simulink library "twiddle_lib"  (Simulink 6.2)
libraries: xbsIndex_r3 x98, coeff_gen_lib x2, twiddle_lib x1
settings Model: LastModifiedBy=aparsons

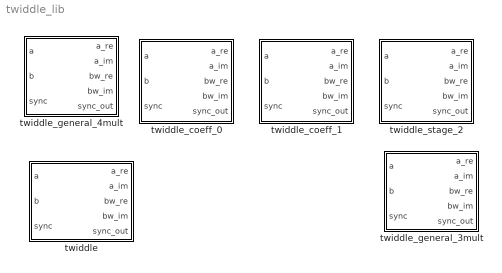
== system twiddle_lib ==
  twiddle : Subsystem  BlockChoice=twiddle_coeff_0
      settings: TemplateBlock=self  MemberBlocks=twiddle_coeff_0,twiddle_coeff_1,twiddle_general_3mult,twiddle_general_4mult,twiddle_stage_2
  twiddle_coeff_0 : Subsystem  mask{BitWidth=18, add_latency=3, mult_latency=4, bram_latency=4}
      mask prompts: BitWidth "Bit Width"; add_latency "Add Latency"; mult_latency "Mult Latency"; bram_latency "BRAM Latency"
      mask init:
      | cursys = gcb;
      | disp(cursys);
  twiddle_coeff_1 : Subsystem  mask{BitWidth=18, add_latency=3, mult_latency=4, bram_latency=4}
      mask prompts: BitWidth "Bit Width"; add_latency "Add Latency"; mult_latency "Mult Latency"; bram_latency "BRAM Latency"
      mask init:
      | cursys = gcb;
      | disp(cursys);
  twiddle_general_3mult : Subsystem  mask{Coeffs=[0], StepPeriod=0, BitWidth=18, add_latency=3, mult_latency=4, bram_latency=4}
      mask prompts: Coeffs "Coefficients:"; StepPeriod "Coefficient Step Period (2^?)"; BitWidth "Bit Width"; add_latency "Add Latency"; mult_latency "Mult Latency"; bram_latency "BRAM Latency"
      mask init:
      | cursys = gcb;
      | disp(cursys);
  twiddle_general_4mult : Subsystem  mask{Coeffs=[0], StepPeriod=0, BitWidth=18, add_latency=3, mult_latency=4, bram_latency=4}
      mask prompts: Coeffs "Coefficients:"; StepPeriod "Coefficient Step Period (2^?)"; BitWidth "Bit Width"; add_latency "Add Latency"; mult_latency "Mult Latency"; bram_latency "BRAM Latency"
      mask init:
      | cursys = gcb;
      | disp(cursys);
  twiddle_stage_2 : Subsystem  mask{FFTSize=5, BitWidth=18, add_latency=3, mult_latency=4, bram_latency=4}
      mask prompts: FFTSize "Size of FFT: (2^?)"; BitWidth "Bit Width"; add_latency "Add Latency"; mult_latency "Mult Latency"; bram_latency "BRAM Latency"
      mask init:
      | cursys = gcb;
      | disp(cursys);

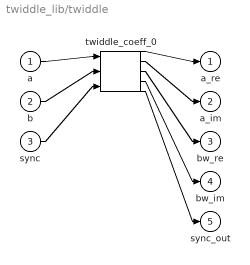
== system twiddle_lib/twiddle ==
  a : Inport  Port=1  LatchInput=off
  b : Inport  Port=2  LatchInput=off
  sync : Inport  Port=3  LatchInput=off
  twiddle_coeff_0 : twiddle_lib/twiddle_coeff_0  BitWidth=18  add_latency=3  mult_latency=4  bram_latency=4
  a_re : Outport
  a_im : Outport  Port=2
  bw_re : Outport  Port=3
  bw_im : Outport  Port=4
  sync_out : Outport  Port=5
  wires:
  a/1 -> twiddle_coeff_0/1
  b/1 -> twiddle_coeff_0/2
  sync/1 -> twiddle_coeff_0/3
  twiddle_coeff_0/1 -> a_re/1
  twiddle_coeff_0/2 -> a_im/1
  twiddle_coeff_0/3 -> bw_re/1
  twiddle_coeff_0/4 -> bw_im/1
  twiddle_coeff_0/5 -> sync_out/1

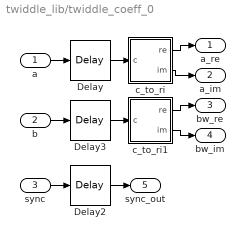
== system twiddle_lib/twiddle_coeff_0 ==
  a : Inport  Port=1  LatchInput=off
  b : Inport  Port=2  LatchInput=off
  sync : Inport  Port=3  LatchInput=off
  Delay : xbsIndex_r3/Delay  latency=mult_latency + add_latency + bram_latency  reg_retiming=off  explicit_period=off  period=1  en=off  accept_only_valid=off  init_zero=on  dbl_ovrd=off  show_param=off
      settings: xl_area=[0, 0, 0, 0, 0, 0, 0]
  Delay2 : xbsIndex_r3/Delay  latency=mult_latency + add_latency + bram_latency  reg_retiming=off  explicit_period=off  period=1  en=off  accept_only_valid=off  init_zero=on  dbl_ovrd=off  show_param=off
      settings: xl_area=[0, 0, 0, 0, 0, 0, 0]
  Delay3 : xbsIndex_r3/Delay  latency=mult_latency + add_latency + bram_latency  reg_retiming=off  explicit_period=off  period=1  en=off  accept_only_valid=off  init_zero=on  dbl_ovrd=off  show_param=off
      settings: xl_area=[0, 0, 0, 0, 0, 0, 0]
  c_to_ri : Subsystem
  c_to_ri1 : Subsystem
  a_re : Outport
  a_im : Outport  Port=2
  bw_re : Outport  Port=3
  bw_im : Outport  Port=4
  sync_out : Outport  Port=5
  wires:
  Delay3/1 -> c_to_ri1/1(c)
  c_to_ri1/2(im) -> bw_im/1
  c_to_ri1/1(re) -> bw_re/1
  c_to_ri/2(im) -> a_im/1
  c_to_ri/1(re) -> a_re/1
  Delay/1 -> c_to_ri/1(c)
  b/1 -> Delay3/1
  Delay2/1 -> sync_out/1
  sync/1 -> Delay2/1
  a/1 -> Delay/1

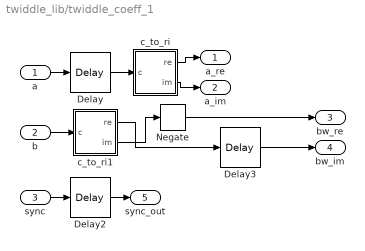
== system twiddle_lib/twiddle_coeff_1 ==
  a : Inport  Port=1  LatchInput=off
  b : Inport  Port=2  LatchInput=off
  sync : Inport  Port=3  LatchInput=off
  Delay : xbsIndex_r3/Delay  latency=mult_latency + add_latency + bram_latency  reg_retiming=off  explicit_period=off  period=1  en=off  accept_only_valid=off  init_zero=on  dbl_ovrd=off  show_param=off
      settings: xl_area=[0, 0, 0, 0, 0, 0, 0]
  Delay2 : xbsIndex_r3/Delay  latency=mult_latency + add_latency + bram_latency  reg_retiming=off  explicit_period=off  period=1  en=off  accept_only_valid=off  init_zero=on  dbl_ovrd=off  show_param=off
      settings: xl_area=[0, 0, 0, 0, 0, 0, 0]
  Delay3 : xbsIndex_r3/Delay  latency=mult_latency + add_latency + bram_latency  reg_retiming=off  explicit_period=off  period=1  en=off  accept_only_valid=off  init_zero=on  dbl_ovrd=off  show_param=off
      settings: xl_area=[0, 0, 0, 0, 0, 0, 0]
  Negate : xbsIndex_r3/Negate  precision=User Defined  arith_type="Signed  (2's comp)"  n_bits=BitWidth  bin_pt=BitWidth-1  quantization=Truncate  overflow=Wrap  latency=mult_latency + add_latency + bram_latency  explicit_period=off  period=1  en=off  dbl_ovrd=off  use_core=on  show_param=off  use_rpm=on  gen_core=off
      settings: xl_area=[0, 0, 0, 0, 0, 0, 0]
  c_to_ri : Subsystem
  c_to_ri1 : Subsystem
  a_re : Outport
  a_im : Outport  Port=2
  bw_re : Outport  Port=3
  bw_im : Outport  Port=4
  sync_out : Outport  Port=5
  wires:
  Delay3/1 -> bw_im/1
  c_to_ri1/2(im) -> Negate/1
  Negate/1 -> bw_re/1
  c_to_ri1/1(re) -> Delay3/1
  a/1 -> Delay/1
  sync/1 -> Delay2/1
  Delay2/1 -> sync_out/1
  b/1 -> c_to_ri1/1(c)
  Delay/1 -> c_to_ri/1(c)
  c_to_ri/1(re) -> a_re/1
  c_to_ri/2(im) -> a_im/1

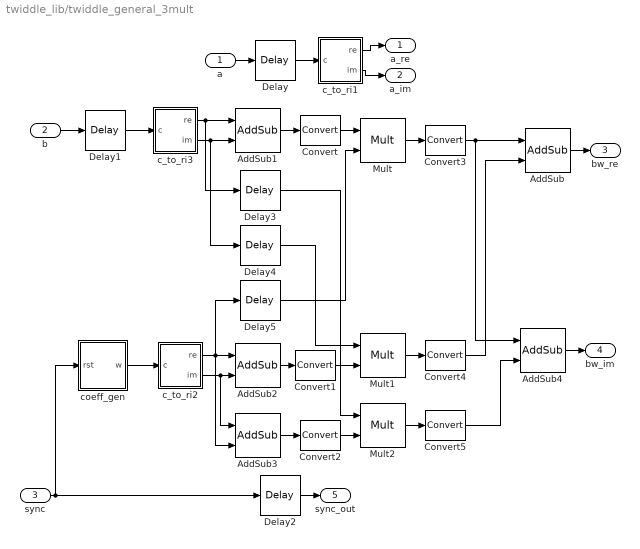
== system twiddle_lib/twiddle_general_3mult ==
  a : Inport  Port=1  LatchInput=off
  b : Inport  Port=2  LatchInput=off
  sync : Inport  Port=3  LatchInput=off
  AddSub : xbsIndex_r3/AddSub  mode=Subtraction  precision=Full  arith_type="Signed  (2's comp)"  n_bits=BitWidth  bin_pt=BitWidth - 1  quantization="Round  (unbiased: +/- Inf)"  overflow=Wrap  latency=add_latency  explicit_period=off  period=1  use_carryin=off  use_carryout=off  en=off  dbl_ovrd=off  show_param=on  use_core=on  pipeline=on  use_rpm=on  gen_core=on
      settings: xl_area=[0, 0, 0, 0, 0, 0, 0]
  AddSub1 : xbsIndex_r3/AddSub  mode=Addition  precision=Full  arith_type="Signed  (2's comp)"  n_bits=BitWidth  bin_pt=BitWidth - 1  quantization="Round  (unbiased: +/- Inf)"  overflow=Wrap  latency=add_latency  explicit_period=off  period=1  use_carryin=off  use_carryout=off  en=off  dbl_ovrd=off  show_param=on  use_core=on  pipeline=on  use_rpm=on  gen_core=on
      settings: xl_area=[0, 0, 0, 0, 0, 0, 0]
  AddSub2 : xbsIndex_r3/AddSub  mode=Addition  precision=Full  arith_type="Signed  (2's comp)"  n_bits=BitWidth  bin_pt=BitWidth - 1  quantization="Round  (unbiased: +/- Inf)"  overflow=Wrap  latency=add_latency  explicit_period=off  period=1  use_carryin=off  use_carryout=off  en=off  dbl_ovrd=off  show_param=on  use_core=on  pipeline=on  use_rpm=on  gen_core=on
      settings: xl_area=[0, 0, 0, 0, 0, 0, 0]
  AddSub3 : xbsIndex_r3/AddSub  mode=Subtraction  precision=Full  arith_type="Signed  (2's comp)"  n_bits=BitWidth  bin_pt=BitWidth - 1  quantization="Round  (unbiased: +/- Inf)"  overflow=Wrap  latency=add_latency  explicit_period=off  period=1  use_carryin=off  use_carryout=off  en=off  dbl_ovrd=off  show_param=on  use_core=on  pipeline=on  use_rpm=on  gen_core=on
      settings: xl_area=[0, 0, 0, 0, 0, 0, 0]
  AddSub4 : xbsIndex_r3/AddSub  mode=Addition  precision=Full  arith_type="Signed  (2's comp)"  n_bits=BitWidth  bin_pt=BitWidth - 1  quantization="Round  (unbiased: +/- Inf)"  overflow=Wrap  latency=add_latency  explicit_period=off  period=1  use_carryin=off  use_carryout=off  en=off  dbl_ovrd=off  show_param=on  use_core=on  pipeline=on  use_rpm=on  gen_core=on
      settings: xl_area=[0, 0, 0, 0, 0, 0, 0]
  Convert : xbsIndex_r3/Convert  arith_type="Signed  (2's comp)"  n_bits=BitWidth  bin_pt=BitWidth-2  quantization=Truncate  overflow=Wrap  latency=0  explicit_period=off  period=1  dbl_ovrd=off  show_param=off  inserted_by_tool=off  pipeline=off
      settings: xl_area=[0, 0, 0, 0, 0, 0, 0]
  Convert1 : xbsIndex_r3/Convert  arith_type="Signed  (2's comp)"  n_bits=BitWidth  bin_pt=BitWidth-2  quantization=Truncate  overflow=Wrap  latency=0  explicit_period=off  period=1  dbl_ovrd=off  show_param=off  inserted_by_tool=off  pipeline=off
      settings: xl_area=[0, 0, 0, 0, 0, 0, 0]
  Convert2 : xbsIndex_r3/Convert  arith_type="Signed  (2's comp)"  n_bits=BitWidth  bin_pt=BitWidth-2  quantization=Truncate  overflow=Wrap  latency=0  explicit_period=off  period=1  dbl_ovrd=off  show_param=off  inserted_by_tool=off  pipeline=off
      settings: xl_area=[0, 0, 0, 0, 0, 0, 0]
  Convert3 : xbsIndex_r3/Convert  arith_type="Signed  (2's comp)"  n_bits=BitWidth + 3  bin_pt=BitWidth  quantization=Truncate  overflow=Wrap  latency=0  explicit_period=off  period=1  dbl_ovrd=off  show_param=off  inserted_by_tool=off  pipeline=off
      settings: xl_area=[0, 0, 0, 0, 0, 0, 0]
  Convert4 : xbsIndex_r3/Convert  arith_type="Signed  (2's comp)"  n_bits=BitWidth + 3  bin_pt=BitWidth  quantization=Truncate  overflow=Wrap  latency=0  explicit_period=off  period=1  dbl_ovrd=off  show_param=off  inserted_by_tool=off  pipeline=off
      settings: xl_area=[0, 0, 0, 0, 0, 0, 0]
  Convert5 : xbsIndex_r3/Convert  arith_type="Signed  (2's comp)"  n_bits=BitWidth + 3  bin_pt=BitWidth  quantization=Truncate  overflow=Wrap  latency=0  explicit_period=off  period=1  dbl_ovrd=off  show_param=off  inserted_by_tool=off  pipeline=off
      settings: xl_area=[0, 0, 0, 0, 0, 0, 0]
  Delay : xbsIndex_r3/Delay  latency=mult_latency + 2*add_latency + bram_latency  reg_retiming=off  explicit_period=off  period=1  en=off  accept_only_valid=off  init_zero=on  dbl_ovrd=off  show_param=off
      settings: xl_area=[0, 0, 0, 0, 0, 0, 0]
  Delay1 : xbsIndex_r3/Delay  latency=bram_latency  reg_retiming=off  explicit_period=off  period=1  en=off  accept_only_valid=off  init_zero=on  dbl_ovrd=off  show_param=off
      settings: xl_area=[0, 0, 0, 0, 0, 0, 0]
  Delay2 : xbsIndex_r3/Delay  latency=mult_latency + 2*add_latency + bram_latency  reg_retiming=off  explicit_period=off  period=1  en=off  accept_only_valid=off  init_zero=on  dbl_ovrd=off  show_param=off
      settings: xl_area=[0, 0, 0, 0, 0, 0, 0]
  Delay3 : xbsIndex_r3/Delay  latency=add_latency  reg_retiming=off  explicit_period=off  period=1  en=off  accept_only_valid=off  init_zero=on  dbl_ovrd=off  show_param=off
      settings: xl_area=[0, 0, 0, 0, 0, 0, 0]
  Delay4 : xbsIndex_r3/Delay  latency=add_latency  reg_retiming=off  explicit_period=off  period=1  en=off  accept_only_valid=off  init_zero=on  dbl_ovrd=off  show_param=off
      settings: xl_area=[0, 0, 0, 0, 0, 0, 0]
  Delay5 : xbsIndex_r3/Delay  latency=add_latency  reg_retiming=off  explicit_period=off  period=1  en=off  accept_only_valid=off  init_zero=on  dbl_ovrd=off  show_param=off
      settings: xl_area=[0, 0, 0, 0, 0, 0, 0]
  Mult : xbsIndex_r3/Mult  precision=Full  arith_type="Signed  (2's comp)"  n_bits=BitWidth  bin_pt=BitWidth-1  quantization="Round  (unbiased: +/- Inf)"  overflow=Wrap  latency=mult_latency  explicit_period=off  period=1  en=off  dbl_ovrd=off  show_param=on  mult_type=Parallel  oversample=2  use_embedded=on  pipeline=on  use_rpm=on  placement_style=Rectangular Shape  gen_core=on
      settings: xl_area=[0, 0, 0, 0, 0, 0, 0]
  Mult1 : xbsIndex_r3/Mult  precision=Full  arith_type="Signed  (2's comp)"  n_bits=BitWidth  bin_pt=BitWidth-1  quantization="Round  (unbiased: +/- Inf)"  overflow=Wrap  latency=mult_latency  explicit_period=off  period=1  en=off  dbl_ovrd=off  show_param=on  mult_type=Parallel  oversample=2  use_embedded=on  pipeline=on  use_rpm=on  placement_style=Rectangular Shape  gen_core=on
      settings: xl_area=[0, 0, 0, 0, 0, 0, 0]
  Mult2 : xbsIndex_r3/Mult  precision=Full  arith_type="Signed  (2's comp)"  n_bits=BitWidth  bin_pt=BitWidth-1  quantization="Round  (unbiased: +/- Inf)"  overflow=Wrap  latency=mult_latency  explicit_period=off  period=1  en=off  dbl_ovrd=off  show_param=on  mult_type=Parallel  oversample=2  use_embedded=on  pipeline=on  use_rpm=on  placement_style=Rectangular Shape  gen_core=on
      settings: xl_area=[0, 0, 0, 0, 0, 0, 0]
  c_to_ri1 : Subsystem
  c_to_ri2 : Subsystem
  c_to_ri3 : Subsystem
  coeff_gen : Subsystem  BlockChoice=static_coeff_gen
      link override br_coeff_gen: Coeffs=Coeffs  StepPeriod=StepPeriod  n_bits=BitWidth  latency=bram_latency
      link override static_coeff_gen: Coeffs=Coeffs  n_bits=BitWidth  latency=bram_latency
      settings: AttributesFormatString=%<BlockChoice>  TemplateBlock=coeff_gen_lib/coeff_gen  MemberBlocks=br_coeff_gen,static_coeff_gen
  a_re : Outport
  a_im : Outport  Port=2
  bw_re : Outport  Port=3
  bw_im : Outport  Port=4
  sync_out : Outport  Port=5
  wires:
  Delay2/1 -> sync_out/1
  sync/1 -> coeff_gen/1(rst), Delay2/1
  a/1 -> Delay/1
  Delay/1 -> c_to_ri1/1(c)
  c_to_ri1/1(re) -> a_re/1
  c_to_ri1/2(im) -> a_im/1
  b/1 -> Delay1/1
  Delay1/1 -> c_to_ri3/1(c)
  coeff_gen/1(w) -> c_to_ri2/1(c)
  c_to_ri3/1(re) -> AddSub1/1, Delay3/1
  c_to_ri3/2(im) -> AddSub1/2, Delay4/1
  c_to_ri2/1(re) -> AddSub2/1, AddSub3/2, Delay5/1
  c_to_ri2/2(im) -> AddSub2/2, AddSub3/1
  AddSub3/1 -> Convert2/1
  AddSub2/1 -> Convert1/1
  AddSub1/1 -> Convert/1
  Convert/1 -> Mult/1
  Convert1/1 -> Mult1/2
  Convert2/1 -> Mult2/2
  Delay4/1 -> Mult1/1
  Delay5/1 -> Mult/2
  Delay3/1 -> Mult2/1
  Mult/1 -> Convert3/1
  Mult1/1 -> Convert4/1
  Mult2/1 -> Convert5/1
  AddSub/1 -> bw_re/1
  AddSub4/1 -> bw_im/1
  Convert3/1 -> AddSub/1, AddSub4/1
  Convert4/1 -> AddSub/2
  Convert5/1 -> AddSub4/2

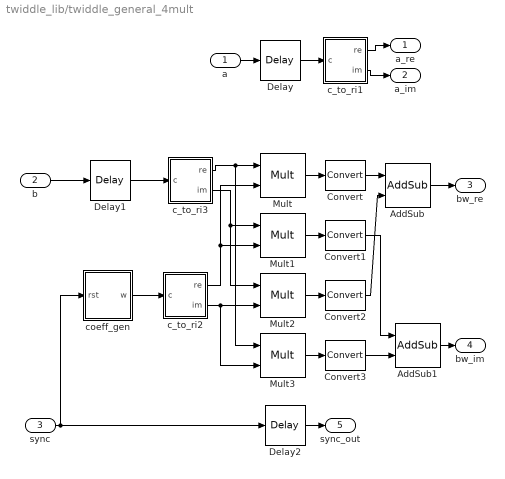
== system twiddle_lib/twiddle_general_4mult ==
  a : Inport  Port=1  LatchInput=off
  b : Inport  Port=2  LatchInput=off
  sync : Inport  Port=3  LatchInput=off
  AddSub : xbsIndex_r3/AddSub  mode=Subtraction  precision=Full  arith_type="Signed  (2's comp)"  n_bits=BitWidth  bin_pt=BitWidth - 1  quantization="Round  (unbiased: +/- Inf)"  overflow=Wrap  latency=add_latency  explicit_period=off  period=1  use_carryin=off  use_carryout=off  en=off  dbl_ovrd=off  show_param=on  use_core=on  pipeline=on  use_rpm=on  gen_core=on
      settings: xl_area=[0, 0, 0, 0, 0, 0, 0]
  AddSub1 : xbsIndex_r3/AddSub  mode=Addition  precision=Full  arith_type="Signed  (2's comp)"  n_bits=BitWidth  bin_pt=BitWidth-1  quantization="Round  (unbiased: +/- Inf)"  overflow=Wrap  latency=add_latency  explicit_period=off  period=1  use_carryin=off  use_carryout=off  en=off  dbl_ovrd=off  show_param=on  use_core=on  pipeline=on  use_rpm=on  gen_core=on
      settings: xl_area=[0, 0, 0, 0, 0, 0, 0]
  Convert{,1..3} (4 alike) : xbsIndex_r3/Convert  arith_type="Signed  (2's comp)"  n_bits=BitWidth + 2  bin_pt=BitWidth  quantization="Round  (unbiased: Even Values)"  overflow=Wrap  latency=0  explicit_period=off  period=1  dbl_ovrd=off  show_param=off  inserted_by_tool=off  pipeline=off
      settings: xl_area=[0, 0, 0, 0, 0, 0, 0]
  Delay : xbsIndex_r3/Delay  latency=mult_latency + add_latency + bram_latency  reg_retiming=off  explicit_period=off  period=1  en=off  accept_only_valid=off  init_zero=on  dbl_ovrd=off  show_param=off
      settings: xl_area=[0, 0, 0, 0, 0, 0, 0]
  Delay1 : xbsIndex_r3/Delay  latency=bram_latency  reg_retiming=off  explicit_period=off  period=1  en=off  accept_only_valid=off  init_zero=on  dbl_ovrd=off  show_param=off
      settings: xl_area=[0, 0, 0, 0, 0, 0, 0]
  Delay2 : xbsIndex_r3/Delay  latency=mult_latency + add_latency + bram_latency  reg_retiming=off  explicit_period=off  period=1  en=off  accept_only_valid=off  init_zero=on  dbl_ovrd=off  show_param=off
      settings: xl_area=[0, 0, 0, 0, 0, 0, 0]
  Mult{,1..3} (4 alike) : xbsIndex_r3/Mult  precision=Full  arith_type="Signed  (2's comp)"  n_bits=BitWidth  bin_pt=BitWidth-1  quantization="Round  (unbiased: +/- Inf)"  overflow=Wrap  latency=mult_latency  explicit_period=off  period=1  en=off  dbl_ovrd=off  show_param=on  mult_type=Parallel  oversample=2  use_embedded=on  pipeline=on  use_rpm=on  placement_style=Rectangular Shape  gen_core=on
      settings: xl_area=[0, 0, 0, 0, 0, 0, 0]
  c_to_ri1 : Subsystem
  c_to_ri2 : Subsystem
  c_to_ri3 : Subsystem
  coeff_gen : Subsystem  BlockChoice=static_coeff_gen
      link override br_coeff_gen: Coeffs=Coeffs  StepPeriod=StepPeriod  n_bits=BitWidth  latency=bram_latency
      link override static_coeff_gen: Coeffs=Coeffs  n_bits=BitWidth  latency=bram_latency
      settings: AttributesFormatString=%<BlockChoice>  TemplateBlock=coeff_gen_lib/coeff_gen  MemberBlocks=br_coeff_gen,static_coeff_gen
  a_re : Outport
  a_im : Outport  Port=2
  bw_re : Outport  Port=3
  bw_im : Outport  Port=4
  sync_out : Outport  Port=5
  wires:
  coeff_gen/1(w) -> c_to_ri2/1(c)
  Delay1/1 -> c_to_ri3/1(c)
  c_to_ri2/2(im) -> Mult3/2, Mult2/2
  c_to_ri3/2(im) -> Mult1/1, Mult2/1
  c_to_ri3/1(re) -> Mult3/1, Mult/1
  b/1 -> Delay1/1
  c_to_ri1/2(im) -> a_im/1
  c_to_ri1/1(re) -> a_re/1
  Delay/1 -> c_to_ri1/1(c)
  AddSub/1 -> bw_re/1
  AddSub1/1 -> bw_im/1
  c_to_ri2/1(re) -> Mult/2, Mult1/2
  Mult/1 -> Convert/1
  Mult2/1 -> Convert2/1
  Mult1/1 -> Convert1/1
  Mult3/1 -> Convert3/1
  a/1 -> Delay/1
  sync/1 -> Delay2/1, coeff_gen/1(rst)
  Delay2/1 -> sync_out/1
  Convert/1 -> AddSub/1
  Convert1/1 -> AddSub1/1
  Convert2/1 -> AddSub/2
  Convert3/1 -> AddSub1/2

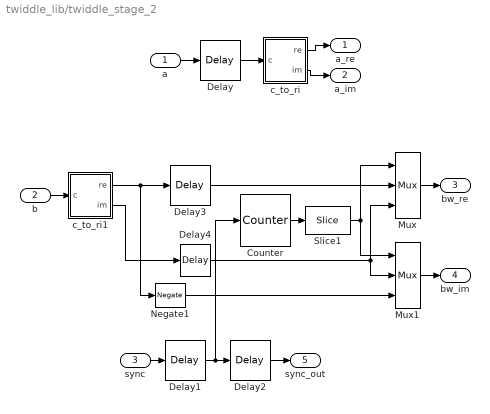
== system twiddle_lib/twiddle_stage_2 ==
  a : Inport  Port=1  LatchInput=off
  b : Inport  Port=2  LatchInput=off
  sync : Inport  Port=3  LatchInput=off
  Counter : xbsIndex_r3/Counter  cnt_type=Free Running  n_bits=FFTSize - 1  bin_pt=0  arith_type=Unsigned  start_count=0  cnt_to=Inf  cnt_by_val=1  operation=Up  explicit_period=off  period=1  load_pin=off  rst=on  en=off  dbl_ovrd=off  show_param=off  use_rpm=on  gen_core=off
      settings: xl_area=[0, 0, 0, 0, 0, 0, 0]
  Delay : xbsIndex_r3/Delay  latency=mult_latency + add_latency + bram_latency  reg_retiming=off  explicit_period=off  period=1  en=off  accept_only_valid=off  init_zero=on  dbl_ovrd=off  show_param=off
      settings: xl_area=[0, 0, 0, 0, 0, 0, 0]
  Delay1 : xbsIndex_r3/Delay  latency=bram_latency  reg_retiming=off  explicit_period=off  period=1  en=off  accept_only_valid=off  init_zero=on  dbl_ovrd=off  show_param=off
      settings: xl_area=[0, 0, 0, 0, 0, 0, 0]
  Delay2 : xbsIndex_r3/Delay  latency=mult_latency + add_latency  reg_retiming=off  explicit_period=off  period=1  en=off  accept_only_valid=off  init_zero=on  dbl_ovrd=off  show_param=off
      settings: xl_area=[0, 0, 0, 0, 0, 0, 0]
  Delay3 : xbsIndex_r3/Delay  latency=bram_latency  reg_retiming=off  explicit_period=off  period=1  en=off  accept_only_valid=off  init_zero=on  dbl_ovrd=off  show_param=off
      settings: xl_area=[0, 0, 0, 0, 0, 0, 0]
  Delay4 : xbsIndex_r3/Delay  latency=bram_latency  reg_retiming=off  explicit_period=off  period=1  en=off  accept_only_valid=off  init_zero=on  dbl_ovrd=off  show_param=off
      settings: xl_area=[0, 0, 0, 0, 0, 0, 0]
  Mux : xbsIndex_r3/Mux  inputs=2  precision=Full  arith_type="Signed  (2's comp)"  n_bits=8  bin_pt=2  quantization=Truncate  overflow=Wrap  latency=mult_latency + add_latency  explicit_period=off  period=1  en=off  dbl_ovrd=off  show_param=off  mux_type=off  use_rpm=off  gen_core=off
      settings: xl_area=[0, 0, 0, 0, 0, 0, 0]
  Mux1 : xbsIndex_r3/Mux  inputs=2  precision=Full  arith_type="Signed  (2's comp)"  n_bits=8  bin_pt=2  quantization=Truncate  overflow=Wrap  latency=mult_latency + add_latency  explicit_period=off  period=1  en=off  dbl_ovrd=off  show_param=off  mux_type=off  use_rpm=off  gen_core=off
      settings: xl_area=[0, 0, 0, 0, 0, 0, 0]
  Negate1 : xbsIndex_r3/Negate  precision=User Defined  arith_type="Signed  (2's comp)"  n_bits=BitWidth  bin_pt=BitWidth-1  quantization=Truncate  overflow=Wrap  latency=bram_latency  explicit_period=off  period=1  en=off  dbl_ovrd=off  use_core=on  show_param=off  use_rpm=on  gen_core=off
      settings: xl_area=[0, 0, 0, 0, 0, 0, 0]
  Slice1 : xbsIndex_r3/Slice  mode=Upper Bit Location + Width  nbits=1  bit1=0  base1=MSB of Input  bit0=0  base0=LSB of Input  boolean_output=off  explicit_period=off  period=1  dbl_ovrd=off
  c_to_ri : Subsystem
  c_to_ri1 : Subsystem
  a_re : Outport
  a_im : Outport  Port=2
  bw_re : Outport  Port=3
  bw_im : Outport  Port=4
  sync_out : Outport  Port=5
  wires:
  Delay4/1 -> Mux/3, Mux1/2
  Delay3/1 -> Mux/2
  Delay1/1 -> Counter/1, Delay2/1
  Mux1/1 -> bw_im/1
  Mux/1 -> bw_re/1
  c_to_ri1/1(re) -> Delay3/1, Negate1/1
  Slice1/1 -> Mux1/1, Mux/1
  Counter/1 -> Slice1/1
  Negate1/1 -> Mux1/3
  c_to_ri1/2(im) -> Delay4/1
  c_to_ri/2(im) -> a_im/1
  c_to_ri/1(re) -> a_re/1
  Delay/1 -> c_to_ri/1(c)
  b/1 -> c_to_ri1/1(c)
  Delay2/1 -> sync_out/1
  sync/1 -> Delay1/1
  a/1 -> Delay/1

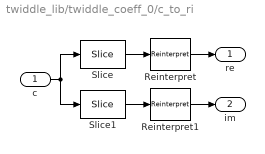
== system twiddle_lib/twiddle_coeff_0/c_to_ri ==
  c : Inport  Port=1  LatchInput=off
  Reinterpret : xbsIndex_r3/Reinterpret  force_arith_type=on  arith_type="Signed  (2's comp)"  force_bin_pt=on  bin_pt=BitWidth - 1  force_valid=on
  Reinterpret1 : xbsIndex_r3/Reinterpret  force_arith_type=on  arith_type="Signed  (2's comp)"  force_bin_pt=on  bin_pt=BitWidth - 1  force_valid=on
  Slice : xbsIndex_r3/Slice  mode=Upper Bit Location + Width  nbits=BitWidth  bit1=0  base1=MSB of Input  bit0=0  base0=LSB of Input  boolean_output=off  explicit_period=off  period=1  dbl_ovrd=off
  Slice1 : xbsIndex_r3/Slice  mode=Lower Bit Location + Width  nbits=BitWidth  bit1=0  base1=MSB of Input  bit0=0  base0=LSB of Input  boolean_output=off  explicit_period=off  period=1  dbl_ovrd=off
  re : Outport
  im : Outport  Port=2
  wires:
  c/1 -> Slice1/1, Slice/1
  Reinterpret1/1 -> im/1
  Reinterpret/1 -> re/1
  Slice1/1 -> Reinterpret1/1
  Slice/1 -> Reinterpret/1

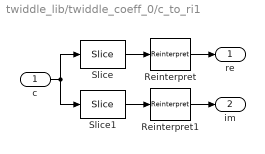
== system twiddle_lib/twiddle_coeff_0/c_to_ri1 ==
  c : Inport  Port=1  LatchInput=off
  Reinterpret : xbsIndex_r3/Reinterpret  force_arith_type=on  arith_type="Signed  (2's comp)"  force_bin_pt=on  bin_pt=BitWidth - 1  force_valid=on
  Reinterpret1 : xbsIndex_r3/Reinterpret  force_arith_type=on  arith_type="Signed  (2's comp)"  force_bin_pt=on  bin_pt=BitWidth - 1  force_valid=on
  Slice : xbsIndex_r3/Slice  mode=Upper Bit Location + Width  nbits=BitWidth  bit1=0  base1=MSB of Input  bit0=0  base0=LSB of Input  boolean_output=off  explicit_period=off  period=1  dbl_ovrd=off
  Slice1 : xbsIndex_r3/Slice  mode=Lower Bit Location + Width  nbits=BitWidth  bit1=0  base1=MSB of Input  bit0=0  base0=LSB of Input  boolean_output=off  explicit_period=off  period=1  dbl_ovrd=off
  re : Outport
  im : Outport  Port=2
  wires:
  c/1 -> Slice1/1, Slice/1
  Reinterpret1/1 -> im/1
  Reinterpret/1 -> re/1
  Slice1/1 -> Reinterpret1/1
  Slice/1 -> Reinterpret/1

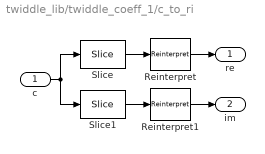
== system twiddle_lib/twiddle_coeff_1/c_to_ri ==
  c : Inport  Port=1  LatchInput=off
  Reinterpret : xbsIndex_r3/Reinterpret  force_arith_type=on  arith_type="Signed  (2's comp)"  force_bin_pt=on  bin_pt=BitWidth - 1  force_valid=on
  Reinterpret1 : xbsIndex_r3/Reinterpret  force_arith_type=on  arith_type="Signed  (2's comp)"  force_bin_pt=on  bin_pt=BitWidth - 1  force_valid=on
  Slice : xbsIndex_r3/Slice  mode=Upper Bit Location + Width  nbits=BitWidth  bit1=0  base1=MSB of Input  bit0=0  base0=LSB of Input  boolean_output=off  explicit_period=off  period=1  dbl_ovrd=off
  Slice1 : xbsIndex_r3/Slice  mode=Lower Bit Location + Width  nbits=BitWidth  bit1=0  base1=MSB of Input  bit0=0  base0=LSB of Input  boolean_output=off  explicit_period=off  period=1  dbl_ovrd=off
  re : Outport
  im : Outport  Port=2
  wires:
  c/1 -> Slice1/1, Slice/1
  Reinterpret1/1 -> im/1
  Reinterpret/1 -> re/1
  Slice1/1 -> Reinterpret1/1
  Slice/1 -> Reinterpret/1

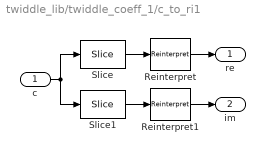
== system twiddle_lib/twiddle_coeff_1/c_to_ri1 ==
  c : Inport  Port=1  LatchInput=off
  Reinterpret : xbsIndex_r3/Reinterpret  force_arith_type=on  arith_type="Signed  (2's comp)"  force_bin_pt=on  bin_pt=BitWidth - 1  force_valid=on
  Reinterpret1 : xbsIndex_r3/Reinterpret  force_arith_type=on  arith_type="Signed  (2's comp)"  force_bin_pt=on  bin_pt=BitWidth - 1  force_valid=on
  Slice : xbsIndex_r3/Slice  mode=Upper Bit Location + Width  nbits=BitWidth  bit1=0  base1=MSB of Input  bit0=0  base0=LSB of Input  boolean_output=off  explicit_period=off  period=1  dbl_ovrd=off
  Slice1 : xbsIndex_r3/Slice  mode=Lower Bit Location + Width  nbits=BitWidth  bit1=0  base1=MSB of Input  bit0=0  base0=LSB of Input  boolean_output=off  explicit_period=off  period=1  dbl_ovrd=off
  re : Outport
  im : Outport  Port=2
  wires:
  c/1 -> Slice1/1, Slice/1
  Reinterpret1/1 -> im/1
  Reinterpret/1 -> re/1
  Slice1/1 -> Reinterpret1/1
  Slice/1 -> Reinterpret/1

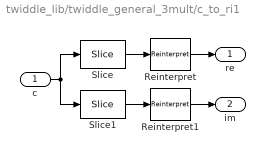
== system twiddle_lib/twiddle_general_3mult/c_to_ri1 ==
  c : Inport  Port=1  LatchInput=off
  Reinterpret : xbsIndex_r3/Reinterpret  force_arith_type=on  arith_type="Signed  (2's comp)"  force_bin_pt=on  bin_pt=BitWidth - 1  force_valid=on
  Reinterpret1 : xbsIndex_r3/Reinterpret  force_arith_type=on  arith_type="Signed  (2's comp)"  force_bin_pt=on  bin_pt=BitWidth - 1  force_valid=on
  Slice : xbsIndex_r3/Slice  mode=Upper Bit Location + Width  nbits=BitWidth  bit1=0  base1=MSB of Input  bit0=0  base0=LSB of Input  boolean_output=off  explicit_period=off  period=1  dbl_ovrd=off
  Slice1 : xbsIndex_r3/Slice  mode=Lower Bit Location + Width  nbits=BitWidth  bit1=0  base1=MSB of Input  bit0=0  base0=LSB of Input  boolean_output=off  explicit_period=off  period=1  dbl_ovrd=off
  re : Outport
  im : Outport  Port=2
  wires:
  Slice/1 -> Reinterpret/1
  Slice1/1 -> Reinterpret1/1
  Reinterpret/1 -> re/1
  Reinterpret1/1 -> im/1
  c/1 -> Slice/1, Slice1/1

== system twiddle_lib/twiddle_general_3mult/c_to_ri2 ==
  c : Inport  Port=1  LatchInput=off
  Reinterpret : xbsIndex_r3/Reinterpret  force_arith_type=on  arith_type="Signed  (2's comp)"  force_bin_pt=on  bin_pt=BitWidth - 1  force_valid=on
  Reinterpret1 : xbsIndex_r3/Reinterpret  force_arith_type=on  arith_type="Signed  (2's comp)"  force_bin_pt=on  bin_pt=BitWidth - 1  force_valid=on
  Slice : xbsIndex_r3/Slice  mode=Upper Bit Location + Width  nbits=BitWidth  bit1=0  base1=MSB of Input  bit0=0  base0=LSB of Input  boolean_output=off  explicit_period=off  period=1  dbl_ovrd=off
  Slice1 : xbsIndex_r3/Slice  mode=Lower Bit Location + Width  nbits=BitWidth  bit1=0  base1=MSB of Input  bit0=0  base0=LSB of Input  boolean_output=off  explicit_period=off  period=1  dbl_ovrd=off
  re : Outport
  im : Outport  Port=2
  wires:
  Slice/1 -> Reinterpret/1
  Slice1/1 -> Reinterpret1/1
  Reinterpret/1 -> re/1
  Reinterpret1/1 -> im/1
  c/1 -> Slice/1, Slice1/1

== system twiddle_lib/twiddle_general_3mult/c_to_ri3 ==
  c : Inport  Port=1  LatchInput=off
  Reinterpret : xbsIndex_r3/Reinterpret  force_arith_type=on  arith_type="Signed  (2's comp)"  force_bin_pt=on  bin_pt=BitWidth - 1  force_valid=on
  Reinterpret1 : xbsIndex_r3/Reinterpret  force_arith_type=on  arith_type="Signed  (2's comp)"  force_bin_pt=on  bin_pt=BitWidth - 1  force_valid=on
  Slice : xbsIndex_r3/Slice  mode=Upper Bit Location + Width  nbits=BitWidth  bit1=0  base1=MSB of Input  bit0=0  base0=LSB of Input  boolean_output=off  explicit_period=off  period=1  dbl_ovrd=off
  Slice1 : xbsIndex_r3/Slice  mode=Lower Bit Location + Width  nbits=BitWidth  bit1=0  base1=MSB of Input  bit0=0  base0=LSB of Input  boolean_output=off  explicit_period=off  period=1  dbl_ovrd=off
  re : Outport
  im : Outport  Port=2
  wires:
  Slice/1 -> Reinterpret/1
  Slice1/1 -> Reinterpret1/1
  Reinterpret/1 -> re/1
  Reinterpret1/1 -> im/1
  c/1 -> Slice/1, Slice1/1

== system twiddle_lib/twiddle_general_3mult/coeff_gen ==
  rst : Inport  Port=1  LatchInput=off
  static_coeff_gen : coeff_gen_lib/static_coeff_gen  Coeffs=Coeffs  n_bits=BitWidth  latency=bram_latency
  w : Outport
  wires:
  rst/1 -> static_coeff_gen/1
  static_coeff_gen/1 -> w/1

== system twiddle_lib/twiddle_general_4mult/c_to_ri1 ==
  c : Inport  Port=1  LatchInput=off
  Reinterpret : xbsIndex_r3/Reinterpret  force_arith_type=on  arith_type="Signed  (2's comp)"  force_bin_pt=on  bin_pt=BitWidth - 1  force_valid=on
  Reinterpret1 : xbsIndex_r3/Reinterpret  force_arith_type=on  arith_type="Signed  (2's comp)"  force_bin_pt=on  bin_pt=BitWidth - 1  force_valid=on
  Slice : xbsIndex_r3/Slice  mode=Upper Bit Location + Width  nbits=BitWidth  bit1=0  base1=MSB of Input  bit0=0  base0=LSB of Input  boolean_output=off  explicit_period=off  period=1  dbl_ovrd=off
  Slice1 : xbsIndex_r3/Slice  mode=Lower Bit Location + Width  nbits=BitWidth  bit1=0  base1=MSB of Input  bit0=0  base0=LSB of Input  boolean_output=off  explicit_period=off  period=1  dbl_ovrd=off
  re : Outport
  im : Outport  Port=2
  wires:
  c/1 -> Slice1/1, Slice/1
  Reinterpret1/1 -> im/1
  Reinterpret/1 -> re/1
  Slice1/1 -> Reinterpret1/1
  Slice/1 -> Reinterpret/1

== system twiddle_lib/twiddle_general_4mult/c_to_ri2 ==
  c : Inport  Port=1  LatchInput=off
  Reinterpret : xbsIndex_r3/Reinterpret  force_arith_type=on  arith_type="Signed  (2's comp)"  force_bin_pt=on  bin_pt=BitWidth - 1  force_valid=on
  Reinterpret1 : xbsIndex_r3/Reinterpret  force_arith_type=on  arith_type="Signed  (2's comp)"  force_bin_pt=on  bin_pt=BitWidth - 1  force_valid=on
  Slice : xbsIndex_r3/Slice  mode=Upper Bit Location + Width  nbits=BitWidth  bit1=0  base1=MSB of Input  bit0=0  base0=LSB of Input  boolean_output=off  explicit_period=off  period=1  dbl_ovrd=off
  Slice1 : xbsIndex_r3/Slice  mode=Lower Bit Location + Width  nbits=BitWidth  bit1=0  base1=MSB of Input  bit0=0  base0=LSB of Input  boolean_output=off  explicit_period=off  period=1  dbl_ovrd=off
  re : Outport
  im : Outport  Port=2
  wires:
  c/1 -> Slice1/1, Slice/1
  Reinterpret1/1 -> im/1
  Reinterpret/1 -> re/1
  Slice1/1 -> Reinterpret1/1
  Slice/1 -> Reinterpret/1

== system twiddle_lib/twiddle_general_4mult/c_to_ri3 ==
  c : Inport  Port=1  LatchInput=off
  Reinterpret : xbsIndex_r3/Reinterpret  force_arith_type=on  arith_type="Signed  (2's comp)"  force_bin_pt=on  bin_pt=BitWidth - 1  force_valid=on
  Reinterpret1 : xbsIndex_r3/Reinterpret  force_arith_type=on  arith_type="Signed  (2's comp)"  force_bin_pt=on  bin_pt=BitWidth - 1  force_valid=on
  Slice : xbsIndex_r3/Slice  mode=Upper Bit Location + Width  nbits=BitWidth  bit1=0  base1=MSB of Input  bit0=0  base0=LSB of Input  boolean_output=off  explicit_period=off  period=1  dbl_ovrd=off
  Slice1 : xbsIndex_r3/Slice  mode=Lower Bit Location + Width  nbits=BitWidth  bit1=0  base1=MSB of Input  bit0=0  base0=LSB of Input  boolean_output=off  explicit_period=off  period=1  dbl_ovrd=off
  re : Outport
  im : Outport  Port=2
  wires:
  c/1 -> Slice1/1, Slice/1
  Reinterpret1/1 -> im/1
  Reinterpret/1 -> re/1
  Slice1/1 -> Reinterpret1/1
  Slice/1 -> Reinterpret/1

== system twiddle_lib/twiddle_general_4mult/coeff_gen ==
  rst : Inport  Port=1  LatchInput=off
  static_coeff_gen : coeff_gen_lib/static_coeff_gen  Coeffs=Coeffs  n_bits=BitWidth  latency=bram_latency
  w : Outport
  wires:
  rst/1 -> static_coeff_gen/1
  static_coeff_gen/1 -> w/1

== system twiddle_lib/twiddle_stage_2/c_to_ri ==
  c : Inport  Port=1  LatchInput=off
  Reinterpret : xbsIndex_r3/Reinterpret  force_arith_type=on  arith_type="Signed  (2's comp)"  force_bin_pt=on  bin_pt=BitWidth - 1  force_valid=on
  Reinterpret1 : xbsIndex_r3/Reinterpret  force_arith_type=on  arith_type="Signed  (2's comp)"  force_bin_pt=on  bin_pt=BitWidth - 1  force_valid=on
  Slice : xbsIndex_r3/Slice  mode=Upper Bit Location + Width  nbits=BitWidth  bit1=0  base1=MSB of Input  bit0=0  base0=LSB of Input  boolean_output=off  explicit_period=off  period=1  dbl_ovrd=off
  Slice1 : xbsIndex_r3/Slice  mode=Lower Bit Location + Width  nbits=BitWidth  bit1=0  base1=MSB of Input  bit0=0  base0=LSB of Input  boolean_output=off  explicit_period=off  period=1  dbl_ovrd=off
  re : Outport
  im : Outport  Port=2
  wires:
  c/1 -> Slice1/1, Slice/1
  Reinterpret1/1 -> im/1
  Reinterpret/1 -> re/1
  Slice1/1 -> Reinterpret1/1
  Slice/1 -> Reinterpret/1

== system twiddle_lib/twiddle_stage_2/c_to_ri1 ==
  c : Inport  Port=1  LatchInput=off
  Reinterpret : xbsIndex_r3/Reinterpret  force_arith_type=on  arith_type="Signed  (2's comp)"  force_bin_pt=on  bin_pt=BitWidth - 1  force_valid=on
  Reinterpret1 : xbsIndex_r3/Reinterpret  force_arith_type=on  arith_type="Signed  (2's comp)"  force_bin_pt=on  bin_pt=BitWidth - 1  force_valid=on
  Slice : xbsIndex_r3/Slice  mode=Upper Bit Location + Width  nbits=BitWidth  bit1=0  base1=MSB of Input  bit0=0  base0=LSB of Input  boolean_output=off  explicit_period=off  period=1  dbl_ovrd=off
  Slice1 : xbsIndex_r3/Slice  mode=Lower Bit Location + Width  nbits=BitWidth  bit1=0  base1=MSB of Input  bit0=0  base0=LSB of Input  boolean_output=off  explicit_period=off  period=1  dbl_ovrd=off
  re : Outport
  im : Outport  Port=2
  wires:
  c/1 -> Slice1/1, Slice/1
  Reinterpret1/1 -> im/1
  Reinterpret/1 -> re/1
  Slice1/1 -> Reinterpret1/1
  Slice/1 -> Reinterpret/1
